simulink model "GalvoModel_v31_no_CC"  (R2013a)
settings: Solver=ode45  StartTime=0.0  StopTime=50e-3  RelTol=1e-3
PreLoadFcn:
  | Kp_cc=evalin('base',paramCtrl.Kp_cc);
InitFcn:
  | Kp_cc=evalin('base',paramCtrl.Kp_cc);
settings Model: BufferReuse=off  Creator=mainster  LastModifiedBy=mainster
settings OptimizationCC: InlineParams=on  BufferReuse=off
settings DebuggingCC: InitInArrayFormatMsg=none
settings ModelReferenceCC: ModelReferenceNumInstancesAllowed=Single

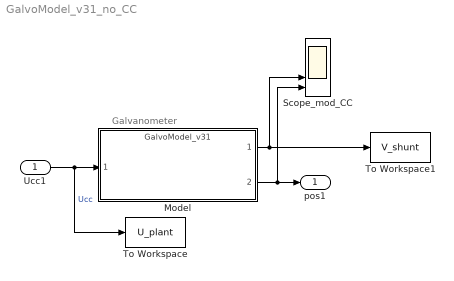
== system GalvoModel_v31_no_CC ==
  note: Galvanometer
  Ucc1 : Inport
  Model : ModelReference  ModelNameDialog=GalvoModel_v31.slx  SimulationMode=Normal  ModelReferenceVersion=1.15  CopyOfModelName=GalvoModel_v31.slx  DefaultDataLogging=on
      mask Display:
      | str=sprintf('%s',get(gcbh,'ModelName'));
      | port_label('input', 1, 'VCoil','texmode','on')
      | color('blue');
      | port_label('output', 1, 'VShunt','texmode','on')
      | color('black');
      | port_label('output', 2, 'AngPos')
      | %text(.05,.98,['{\fontsize{12}\it\bf' strrep(str,'_',' ') '}'],'horizontalAlignment','left','verticalAlignment','top','texmode','on')
      | text(.05,.98,['{\fontsize{12}\it\bf' strrep(str,'_','\_') '}'],'horizontalAlignment','left','verticalAlignment','top','texmode','on')
      | 
      | %get_param(gcbh,'Location')
      | % pos = get_param(gcb, 'Position');
      | % width = pos(3) - pos(1);
      | % x = [0, width];
      | % y = ones(1,length(x))*0.8;
      | % plot(x,y)
  Scope_mod_CC : Scope  NumInputPorts=5
      settings: ShowLegends=on  TimeRange=0.03  YMin=-1~-1~-1~-0.02~0  YMax=3~3~3~0.06~0.02  MaxDataPoints=500000
  To Workspace : ToWorkspace  VariableName=U_plant  SampleTime=-1  SaveFormat=Timeseries
  To Workspace1 : ToWorkspace  VariableName=V_shunt  SampleTime=-1  SaveFormat=Timeseries
  pos1 : Outport
  wires:
  Model/2 -> Scope_mod_CC/5, pos1/1
  Ucc1/1 -> To Workspace/1, Model/1  "Ucc"
  Model/1 -> To Workspace1/1, Scope_mod_CC/4
